simulink model "WGmodel_v3"  (R2022b)
settings: Solver=VariableStepAuto  StartTime=0.0  StopTime=5  MinStep=1e-3  RelTol=1e-3
values from neighbouring files (symbols this model uses):
  pinitwindgen = 0.5161    [WGmodel_startup.m]    (also in WGmodel_startup_v2.m; WGmodel_startup_v3.m = pinitwindgen(1))
  R = 0.05    [WGmodel_startup.m]    (also in WGmodel_startup_v2.m; WGmodel_startup_v3.m)
  tableData = []    [LUT_2D.m]
  Tc2 = 0.05    [WGmodel_startup.m]    (also in WGmodel_startup_v2.m; WGmodel_startup_v3.m)
  v_beta = 0:1:2    [WGmodel_startup.m]    (also in fun_getwindpowercurve_v2.m = 0.5)
  v_vw = 5:10    [LUT_2D.m]    (also in WGmodel_startup.m = 5:1:10; WGmodel_startup_v2.m = 5:1:15; WGmodel_startup_v3.m = 5:.5:12; fun_getwindpowercurve_v2.m = [10 11 12])
  v_wr = v_Wr/Wrn    [fun_getwindpowercurve.m]    (also in fun_getwindpowercurve_v2.m; fun_getwindpowercurve_v3.m; fun_getwindpowercurve_v4.m; fun_getwindpowercurve_v5.m)
libraries: slpidlib x1
settings Model: Creator=User  LastModifiedBy=User
settings DataIOCC: ReturnWorkspaceOutputsName=tpca2c73f9_aaf2_4561_a91a_5350207c853f

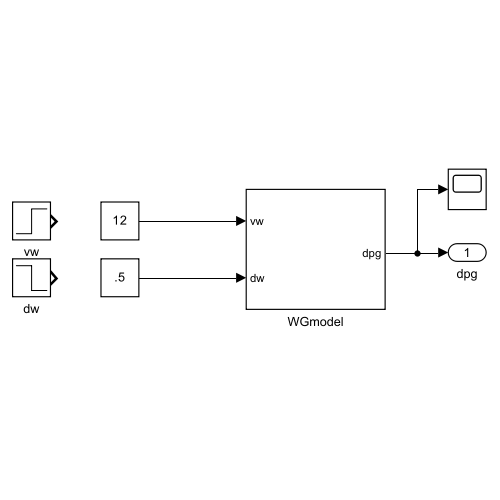
[thumbnail: Simulink's stored preview of the top-level diagram]
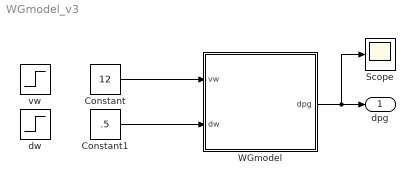
== system WGmodel_v3 ==
  Constant : Constant  Value=12
  Constant1 : Constant  Value=.5
  Scope : Scope
  WGmodel : Subsystem
  dw : Step  After=-0.5  SampleTime=0
  vw : Step  After=10  SampleTime=0
  dpg : Outport  VectorParamsAs1DForOutWhenUnconnected=off
  wires:
  WGmodel/1(dpg) -> Scope/1, dpg/1
  Constant/1 -> WGmodel/1(vw)
  Constant1/1 -> WGmodel/2(dw)

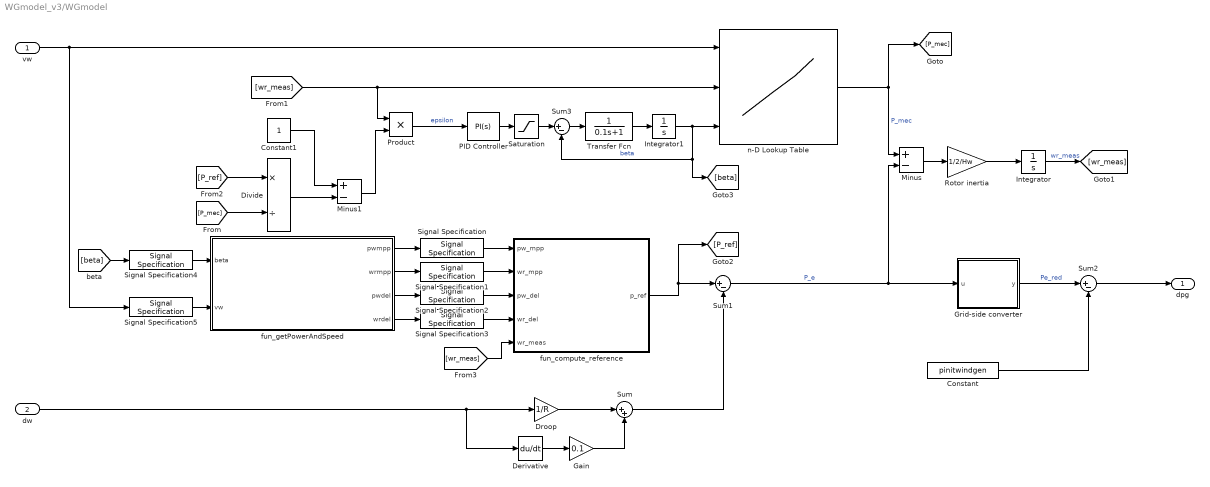
== system WGmodel_v3/WGmodel ==
  vw : Inport
  dw : Inport  Port=2
  Constant : Constant  Value=pinitwindgen
  Constant1 : Constant
  Derivative : Derivative
  Divide : Product  Inputs=*/
  Droop : Gain  Gain=1/R
  Gain : Gain  Gain=0.1
  Grid-side converter : Subsystem  mask{T=Tc2, y0=pinitwindgen}
      mask prompts: T "Time constant (s)"; y0 "Initial condition (pu)"
  Integrator : Integrator  InitialCondition=1
  Integrator1 : Integrator
  Minus : Sum  Inputs=+-
  Minus1 : Sum  Inputs=+-
  PID Controller : slpidlib/PID Controller  Controller=PI  Form=Parallel  TimeDomain=Continuous-time  UseExternalTs=off  SampleTime=-1  IntegratorMethod=Forward Euler  FilterMethod=Forward Euler  ControllerParametersSource=internal  P=355  I=0.01  UseKiTs=off  D=0  N=100  UseFilter=on  TunerSelectOption=Transfer Function Based (PID Tuner App)  InitialConditionSource=internal  InitialConditionForIntegrator=0  InitialConditionForFilter=0  DifferentiatorICPrevScaledInput=0  ExternalReset=none  TrackingMode=off  Kt=1  LimitOutput=off  SatLimitsSource=internal  UpperSaturationLimit=inf  LowerSaturationLimit=-inf  LinearizeAsGain=on  AntiWindupMode=none  Kb=1  LimitIntegrator=off  UpperIntegratorSaturationLimit=inf  LowerIntegratorSaturationLimit=-inf  POutMin=[]  POutMax=[]  IOutMin=[]  IOutMax=[]  DOutMin=[]  DOutMax=[]  NOutMin=[]  NOutMax=[]  SumOutMin=[]  SumOutMax=[]  SaturationOutMin=[]  SaturationOutMax=[]  PParamMin=[]  PParamMax=[]  IParamMin=[]  IParamMax=[]  DParamMin=[]  DParamMax=[]  NParamMin=[]  NParamMax=[]  KbParamMin=[]  KbParamMax=[]  KtParamMin=[]  KtParamMax=[]  KbOutMin=[]  KbOutMax=[]  KtOutMin=[]  KtOutMax=[]  IntegratorOutMin=[]  IntegratorOutMax=[]  FilterOutMin=[]  FilterOutMax=[]  SumI1OutMin=[]  SumI1OutMax=[]  SumI2OutMin=[]  SumI2OutMax=[]  SumI3OutMin=[]  SumI3OutMax=[]  SumI4OutMin=[]  SumI4OutMax=[]  SumDOutMin=[]  SumDOutMax=[]  DifferentiatorOutMin=[]  DifferentiatorOutMax=[]  FilterDiffOutCoefMin=[]  FilterDiffOutCoefMax=[]  ReciprocalOutMin=[]  ReciprocalOutMax=[]  SumDenOutMin=[]  SumDenOutMax=[]  SumNumOutMin=[]  SumNumOutMax=[]  DivideOutMin=[]  DivideOutMax=[]  UdiffTsProdOutMin=[]  UdiffTsProdOutMax=[]  NTsProdOutMin=[]  NTsProdOutMax=[]  UintegralTsProdOutMin=[]  UintegralTsProdOutMax=[]  UngainTsProdOutMin=[]  UngainTsProdOutMax=[]  ClampingZeroOutDataTypeStr=Inherit: Inherit via back propagation  ClampingZeroOutMin=[]  ClampingZeroOutMax=[]  FilterDenConstantOutDataTypeStr=Inherit: Inherit via back propagation  FilterDenConstantOutMin=[]  FilterDenConstantOutMax=[]  PCopyOutDataTypeStr=Inherit: Inherit via back propagation  PCopyOutMin=[]  PCopyOutMax=[]  NCopyOutDataTypeStr=Inherit: Inherit via back propagation  NCopyOutMin=[]  NCopyOutMax=[]  IntegratorContinuousStateAttributes=''  IntegratorStateMustResolveToSignalObject=off  IntegratorRTWStateStorageClass=Auto  FilterContinuousStateAttributes=''  FilterStateMustResolveToSignalObject=off  FilterRTWStateStorageClass=Auto  ParallelPVariant=InternalParameters  IdealPVariant=Disabled  IVariant=InternalParameters  DVariant=Disabled  IntegratorVariant=Continuous  SatVariant=Disabled  AWVariant=Passthrough  PCopyVariant=Disabled  TRVariant=Disabled  FdbkBlocksVariant=Forward  IdealPFdbkVariant=Disabled  SatFdbkVariant=Disabled  DerivativeFilterVariant=Disabled  NVariant=Disabled  NCopyVariant=Disabled_SignalSpec  FilterICVariant=Disabled  IntegratorICVariant=InternalICs  ExternalResetVariant=Disabled  TRSumVariant=Passthrough  SumFdbkVariant=Disabled  SumVariant=Sum_PI  TsampFilterVariant=InternalTs  TsampNgainVariant=Passthrough  TsampIntegralVariant=Passthrough  ExternalSaturationOutDataTypeStr=Inherit: Same as second input
  Product : Product
  Rotor inertia : Gain  Gain=1/2/Hw
  Saturation : Saturate
  Signal Specification{,1..5} (6 alike) : SignalSpecification  OutDataTypeStr=double
  Sum : Sum  Inputs=|++
  Sum1 : Sum  Inputs=|+-
  Sum2 : Sum  Inputs=|+-
  Sum3 : Sum  Inputs=|+-
  Transfer Fcn : TransferFcn  Denominator=[0.1 1]
  fun_compute_reference : MATLAB Function  TreatAsAtomicUnit=on
  fun_getPowerAndSpeed : MATLAB Function  TreatAsAtomicUnit=on
  n-D Lookup Table : Lookup_n-D  NumberOfTableDimensions=3  BreakpointsForDimension1=v_vw  BreakpointsForDimension2=v_wr  BreakpointsForDimension3=v_beta  Table=tableData  InternalRulePriority=Speed  RndMeth=Simplest
      settings: InputPortMap=u0,u1,u2
  dpg : Outport
  wires:
  Grid-side converter/1(y) -> Sum2/1  "Pe_red"
  Product/1 -> PID Controller/1  "epsilon"
  Saturation/1 -> Sum3/1
  Integrator1/1 -> [beta], Sum3/2, n-D Lookup Table/3  "beta"
  vw/1 -> n-D Lookup Table/1, Signal Specification5/1
  fun_compute_reference/1(p_ref) -> [P_ref], Sum1/1
  [wr_meas] -> Product/1, n-D Lookup Table/2
  Sum1/1 -> Grid-side converter/1(u), Minus/2  "P_e"
  Sum2/1 -> dpg/1
  Minus1/1 -> Product/2
  Minus/1 -> Rotor inertia/1
  Transfer Fcn/1 -> Integrator1/1
  [wr_meas] -> fun_compute_reference/5(wr_meas)
  Constant1/1 -> Minus1/1
  Gain/1 -> Sum/2
  PID Controller/1 -> Saturation/1
  Rotor inertia/1 -> Integrator/1
  n-D Lookup Table/1 -> [P_mec], Minus/1  "P_mec"
  dw/1 -> Derivative/1, Droop/1
  [P_ref] -> Divide/1
  [P_mec] -> Divide/2
  Integrator/1 -> [wr_meas]  "wr_meas"
  Divide/1 -> Minus1/2
  Droop/1 -> Sum/1
  Derivative/1 -> Gain/1
  Sum/1 -> Sum1/2
  Sum3/1 -> Transfer Fcn/1
  Constant/1 -> Sum2/2
  Signal Specification/1 -> fun_compute_reference/1(pw_mpp)
  fun_getPowerAndSpeed/2(wrmpp) -> Signal Specification1/1
  fun_getPowerAndSpeed/4(wrdel) -> Signal Specification3/1
  fun_getPowerAndSpeed/3(pwdel) -> Signal Specification2/1
  fun_getPowerAndSpeed/1(pwmpp) -> Signal Specification/1
  Signal Specification1/1 -> fun_compute_reference/2(wr_mpp)
  Signal Specification2/1 -> fun_compute_reference/3(pw_del)
  Signal Specification3/1 -> fun_compute_reference/4(wr_del)
  [beta] -> Signal Specification4/1
  Signal Specification4/1 -> fun_getPowerAndSpeed/1(beta)
  Signal Specification5/1 -> fun_getPowerAndSpeed/2(vw)

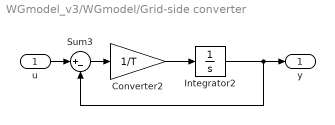
== system WGmodel_v3/WGmodel/Grid-side converter ==
  u : Inport
  Converter2 : Gain  Gain=1/T
  Integrator2 : Integrator  InitialCondition=y0
  Sum3 : Sum  Inputs=|+-
  y : Outport
  wires:
  Integrator2/1 -> y/1, Sum3/2
  Sum3/1 -> Converter2/1
  Converter2/1 -> Integrator2/1
  u/1 -> Sum3/1

== matlab function WGmodel_v3/WGmodel/fun_compute_reference ==
  data: pw_mpp input; p_ref output double size=1; wr_mpp input; pw_del input; wr_del input; wr_meas input
function p_ref = fun_compute_reference(pw_mpp, wr_mpp, pw_del, wr_del, wr_meas)

p_ref = pw_del + (pw_mpp - pw_del)*(wr_del - wr_meas)/(wr_del - wr_mpp);

== matlab function WGmodel_v3/WGmodel/fun_getPowerAndSpeed ==
  data: beta input; pwmpp output; vw input; wrmpp output; pwdel output; wrdel output
function [pwmpp,wrmpp,pwdel,wrdel] = fun_getwindpowercurve_v5(beta,vw)

% This newer version uses scalar values as inputs, rather than vectors.
% The MPP and deloaded outputs are also scalar, not vectors.

% This function computes the power-speed curves for wind generation.
% The power-speed curve of a 1.5 MW wind generator is used for this
% purpose. The resulting curve must be appropriately scaled.
%
% Input:    angle of attack, beta, and wind speed, vw
% Output:   wind power, pw, rotor speed, wr, MPP power, pwmpp, MPP rotor
%           speed, wrmpp

deload = 0.1; % percentage of deloading
rho = 1.275; % air density

% 1.5 MW wind generator data
Rb = 31.2; % blade radius (m)
Aw = Rb^2*pi; % surface 
Pn = 1.5e6; % nominal power (MW)
v_cp = [0.73, 151, 0.58, 0.002, 2.14, 13.2, 18.4, -0.02, -0.003]; % performance coefficients
v_Wr = 0:0.01:4; % rotor speed range (rad/s)

nwr = length(v_Wr);

v_pw    = zeros(1,nwr);
v_wr    = zeros(1,nwr);
pwmpp = 0;
wrmpp = 0;
pwdel = 0;
wrdel = 0;
iwrmpp= 0;

lambda = v_Wr*Rb./vw;
delta = (1./(lambda+v_cp(8).*beta)-v_cp(9)./(1+beta.^3));
Cp = v_cp(1)*(v_cp(2).*delta-v_cp(3).*beta-v_cp(4).*beta.^v_cp(5)-v_cp(6)).*exp(-v_cp(7).*delta);
v_pw(:) = Cp*rho/2*Aw*vw.^3/Pn; % per unit mechanical power

[pwmpp,iwrmpp] = max(v_pw); % MPP
pwdel = (1-deload) * pwmpp; % deloaded

% ==> Algorithm to obtain deloaded speed and power:
% Look up for the "0.9*max(m_pw,[],2)" value (in other words, pw_del) and
% see its corresponding i. Then we look for the corresponding wr value with
% that i.

iwrdel= 0;
wrdel = 0;
Wrdel = 0;

% look for the value closest to pw_del on the right hand side of pmax and
% take note of the index. Then obtain the associated wr

% it takes the right half of the curve after the corresponding MPP point
% and gets it index of the deloaded power
[~,iwrdel] = min(abs(v_pw(iwrmpp:end) - pwdel));
Wrdel    = v_Wr(iwrmpp+iwrdel); % gives the corresponding wr

% ipwmppn = find(v_pwmpp<=1,1,'last'); % nominal power (1 pu)
%ipwmppn = iwrmpp; % nominal power (1 pu)
Wrn = v_Wr(iwrmpp); % nominal speed
v_wr = v_Wr/Wrn;
%v_wr = v_Wr;

Wrmpp = v_Wr(iwrmpp);
wrmpp = Wrmpp/Wrn; % speed corresponding to MPP
wrdel = Wrdel/Wrn; % speed corresponding to deloaded operation points

% figure(1)
% plot(v_wr,v_pw',':b');hold on;
% plot(wrmpp,pwmpp,'-o');hold on;
% plot(wrdel,pwdel,'-o');hold off;
